simulink model "RLCcktStepResponse"  (R2013a)
settings: Solver=ode45  StartTime=0.0  StopTime=0.0000009  MaxStep=1e-4  RelTol=1e-5
libraries: powerlib x9
settings Model: Creator=hp  LastModifiedBy=hp

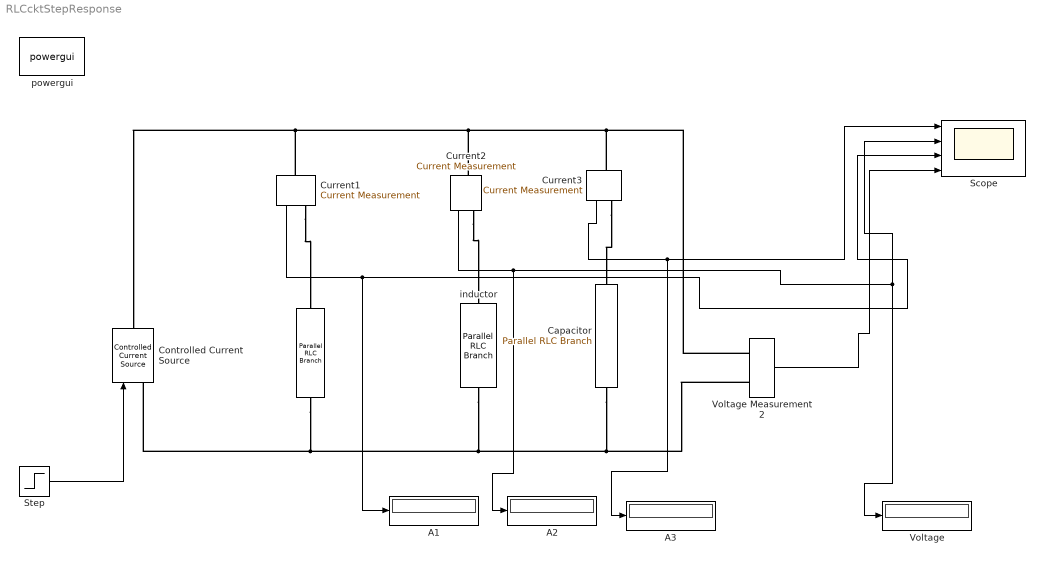
== system RLCcktStepResponse ==
  " " : powerlib/Elements/Parallel RLC Branch  LConnTagsString=a  RConnTagsString=__new0  BranchType=R  Resistance=20  Inductance=1e-3  SetiL0=off  InitialCurrent=0  Capacitance=1e-6  Setx0=off  InitialVoltage=0  Measurements=None
  A1 : Display
  A2 : Display
  A3 : Display
  Capacitor : powerlib/Elements/Parallel RLC Branch  LConnTagsString=a  RConnTagsString=__new0  BranchType=C  Resistance=1  Inductance=1e-3  SetiL0=off  InitialCurrent=0  Capacitance=0.10e-6  Setx0=off  InitialVoltage=0  Measurements=None
  Controlled Current Source : powerlib/Electrical Sources/Controlled Current Source  Initialize=on  Source_Type=AC  Amplitude=0  Phase=0  Frequency=0  Measurements=None
  Current1 : powerlib/Measurements/Current Measurement  PhasorSimulation=off  OutputType=Complex  PSBequivalent=0
  "Current2 " : powerlib/Measurements/Current Measurement  PhasorSimulation=off  OutputType=Complex  PSBequivalent=0
  "Current3 " : powerlib/Measurements/Current Measurement  PhasorSimulation=off  OutputType=Complex  PSBequivalent=0
  Scope : Scope  NumInputPorts=4
      settings: YMin=-5~-5~-5~-5  YMax=5~5~5~5  SaveName=sc
  Step : Step  Before=-2  After=2  SampleTime=0
  "Voltage " : Display
  Voltage Measurement2 : powerlib/Measurements/Voltage Measurement  PhasorSimulation=off  OutputType=Complex  PSBequivalent=0
  inductor : powerlib/Elements/Parallel RLC Branch  LConnTagsString=a  RConnTagsString=__new0  BranchType=L  Resistance=1  Inductance=2e-3  SetiL0=off  InitialCurrent=0  Capacitance=1e-6  Setx0=off  InitialVoltage=0  Measurements=None
  powergui : powerlib/powergui  Priority=1  SimulationMode=Continuous  SolverType=Tustin  SampleTime=50e-6  frequency=60  SPID=off  DisableSnubberDevices=off  DisableRonSwitches=off  DisableVfSwitches=off  SwTol=0  Interpol=off  DisplayEquations=off  frequencyindice=0  Pbase=100e6  ErrMax=1e-4  Iterations=50  UnitsV=kV  UnitsW=MW  FunctionMessages=off  echomessages=off  HookPort=off  EnableUseOfTLC=off  x0status=blocks  RestoreLinks=warning  ResistiveCurrentMeasurement=off  Frange=[0:2:500]  Ylog=off  Xlog=on  ShowGrid=off  save=off  variable=ZData  ZoomFFT=off  StartTime=0.0  cycles=1  DisplayStyle=1  fundamental=60  FreqAxis=off  MaxFrequency=1000  frequencyindicesteady=1  RmsSteady=1  display=off  Ts=0  methode=off
  wires:
  Step/1 -> Controlled Current Source/1
  "Current3 "/1 -> A3/1, Scope/1
  "Current2 "/1 -> A2/1, "Voltage "/1, Scope/2
  Current1/1 -> A1/1, Scope/3
  Voltage Measurement2/1 -> Scope/4
  connections:
  Current1/LConn1 -- "Current3 "/LConn1 -- Voltage Measurement2/LConn1 -- "Current2 "/LConn1 -- Controlled Current Source/RConn1
  inductor/RConn1 -- Voltage Measurement2/LConn2 -- Capacitor/RConn1 -- Controlled Current Source/LConn1 -- " "/RConn1
  Current1/RConn1 -- " "/LConn1
  "Current2 "/RConn1 -- inductor/LConn1
  "Current3 "/RConn1 -- Capacitor/LConn1
